simulink model "EMB_M17"  (R2017b)
settings: Solver=VariableStepAuto  StartTime=0.0  StopTime=10.0  RelTol=1e-3
undefined symbols (not defined in the file): a, b, c_break, c_gear, D_Kraft, D_Pos, d_rot, d_trans, i, I_Kraft, I_Pos, J, K, L, m, P_Kraft, P_Pos, R, t0, t1, T_abtast, x0, x_break
libraries: simulink x4

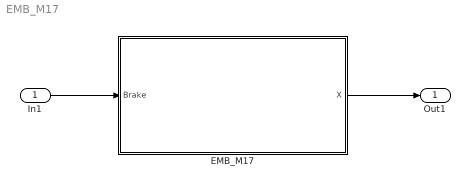
== system EMB_M17 ==
  In1 : Inport
  EMB_M17 : Subsystem
  Out1 : Outport
  wires:
  EMB_M17/1(X) -> Out1/1
  In1/1 -> EMB_M17/1(Brake)

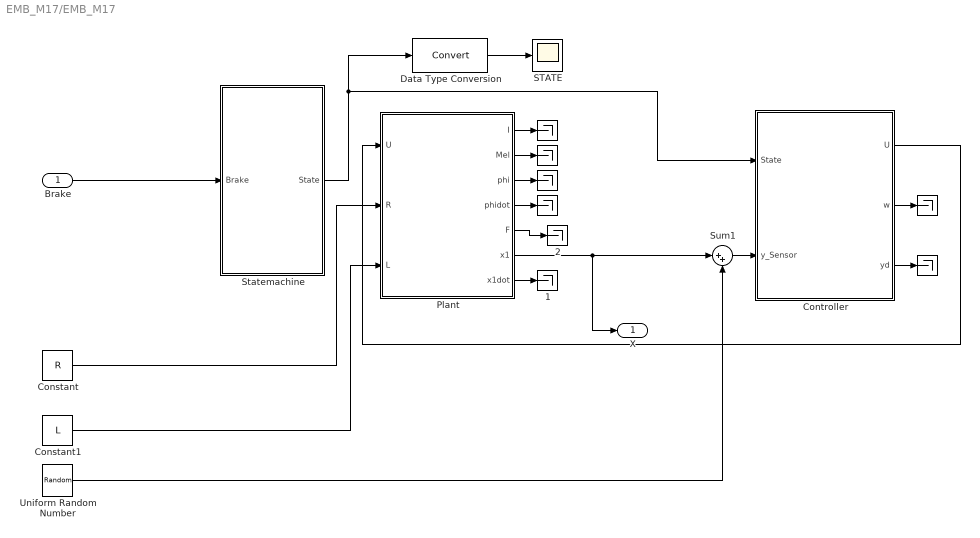
== system EMB_M17/EMB_M17 ==
  Brake : Inport
  "  " : Terminator
  "   " : Terminator
  "    " : Terminator
  "      " : Terminator
  "        " : Terminator
  "          " : Terminator
  "   1" : Terminator
  "   2" : Terminator
  Constant : Constant  Value=R
  Constant1 : Constant  Value=L
  Controller : Subsystem
  Data Type Conversion : DataTypeConversion
  Plant : Subsystem
  STATE : Scope
  Statemachine : Subsystem
  Sum1 : Sum  Inputs=|++
  Uniform Random Number : UniformRandomNumber  Minimum=-0.05  Maximum=0.05  SampleTime=0.000005
  X : Outport
  wires:
  Constant1/1 -> Plant/3(L)
  Constant/1 -> Plant/2(R)
  Data Type Conversion/1 -> STATE/1
  Statemachine/1(State) -> Data Type Conversion/1, Controller/1(State)
  Controller/3(yd) -> "        "/1
  Controller/2(w) -> "          "/1
  Controller/1(U) -> Plant/1(U)
  Sum1/1 -> Controller/2(y_Sensor)
  Plant/1(I) -> "      "/1
  Plant/2(Mel) -> "    "/1
  Uniform Random Number/1 -> Sum1/2
  Plant/7(x1dot) -> "   1"/1
  Plant/5(F) -> "   2"/1
  Plant/4(phidot) -> "   "/1
  Plant/3(phi) -> "  "/1
  Plant/6(x1) -> Sum1/1, X/1
  Brake/1 -> Statemachine/1(Brake)

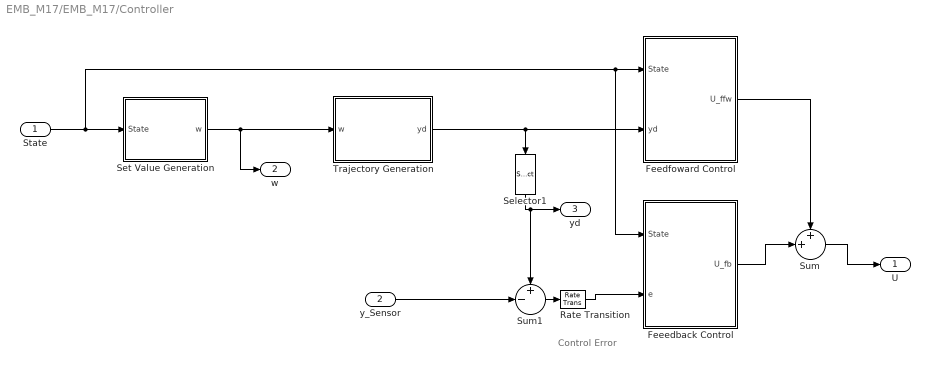
== system EMB_M17/EMB_M17/Controller ==
  note: Control Error
  State : Inport
  y_Sensor : Inport  Port=2
  Feedfoward Control : Subsystem
  Feeedback Control : Subsystem
  Rate Transition : RateTransition
  Selector1 : Selector  InputPortWidth=6  IndexOptions=Index vector (dialog)  Indices=[1]  OutputSizes=1
  Set Value Generation : Subsystem
  Sum : Sum  Inputs=++|
  Sum1 : Sum  Inputs=+-|
  Trajectory Generation : Subsystem
  U : Outport
  w : Outport  Port=2
  yd : Outport  Port=3
  wires:
  Rate Transition/1 -> Feeedback Control/2(e)
  y_Sensor/1 -> Sum1/2
  Selector1/1 -> yd/1, Sum1/1
  Sum1/1 -> Rate Transition/1
  Feeedback Control/1(U_fb) -> Sum/2
  Sum/1 -> U/1
  Feedfoward Control/1(U_ffw) -> Sum/1
  Trajectory Generation/1(yd) -> Selector1/1, Feedfoward Control/2(yd)
  Set Value Generation/1(w) -> w/1, Trajectory Generation/1(w)
  State/1 -> Feeedback Control/1(State), Feedfoward Control/1(State), Set Value Generation/1(State)

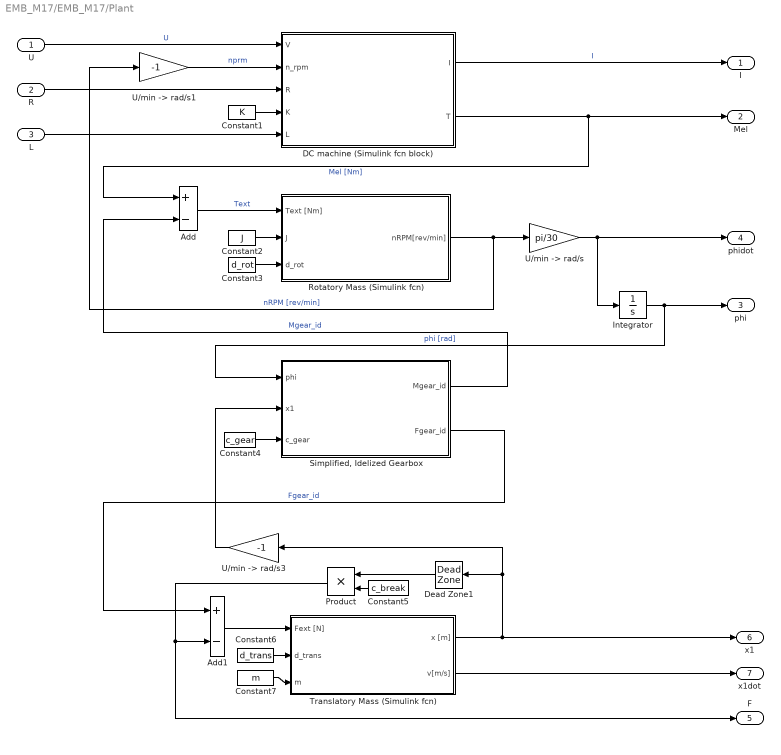
== system EMB_M17/EMB_M17/Plant ==
  U : Inport
  R : Inport  Port=2
  L : Inport  Port=3
  Add : Sum  Inputs=+-
  Add1 : Sum  Inputs=+-
  Constant1 : Constant  Value=K
  Constant2 : Constant  Value=J
  Constant3 : Constant  Value=d_rot
  Constant4 : Constant  Value=c_gear
  Constant5 : Constant  Value=c_break
  Constant6 : Constant  Value=d_trans
  Constant7 : Constant  Value=m
  DC machine (Simulink fcn block) : Subsystem
  Dead Zone1 : DeadZone  LowerValue=-inf  UpperValue=x0  SaturateOnIntegerOverflow=on
  Integrator : Integrator
  Product : Product
  Rotatory Mass (Simulink fcn) : Subsystem
  "Simplified, Idelized Gearbox" : Subsystem
  Translatory Mass (Simulink fcn) : Subsystem
  "U/min -> rad/s" : Gain  Gain=pi/30
  "U/min -> rad/s1" : Gain  Gain=-1
  "U/min -> rad/s3" : Gain  Gain=-1
  I : Outport
  Mel : Outport  Port=2
  phi : Outport  Port=3
  phidot : Outport  Port=4
  F : Outport  Port=5
  x1 : Outport  Port=6
  x1dot : Outport  Port=7
  wires:
  Constant7/1 -> Translatory Mass (Simulink fcn)/3(m)
  Constant6/1 -> Translatory Mass (Simulink fcn)/2(d_trans)
  Constant5/1 -> Product/2
  Constant4/1 -> "Simplified, Idelized Gearbox"/3(c_gear)
  Constant3/1 -> Rotatory Mass (Simulink fcn)/3(d_rot)
  Constant2/1 -> Rotatory Mass (Simulink fcn)/2(J)
  L/1 -> DC machine (Simulink fcn block)/5(L)
  Constant1/1 -> DC machine (Simulink fcn block)/4(K)
  R/1 -> DC machine (Simulink fcn block)/3(R)
  Translatory Mass (Simulink fcn)/2(v[m/s]) -> x1dot/1
  DC machine (Simulink fcn block)/1(I) -> I/1  "I"
  Add/1 -> Rotatory Mass (Simulink fcn)/1(Text [Nm])  "Text"
  Rotatory Mass (Simulink fcn)/1(nRPM[rev/min]) -> "U/min -> rad/s1"/1, "U/min -> rad/s"/1  "nRPM [rev/min]"
  "U/min -> rad/s"/1 -> phidot/1, Integrator/1
  Integrator/1 -> "Simplified, Idelized Gearbox"/1(phi), phi/1  "phi [rad]"
  Add1/1 -> Translatory Mass (Simulink fcn)/1(Fext [N])
  Translatory Mass (Simulink fcn)/1(x [m]) -> x1/1, "U/min -> rad/s3"/1, Dead Zone1/1
  DC machine (Simulink fcn block)/2(T) -> Add/1, Mel/1  "Mel [Nm]"
  "Simplified, Idelized Gearbox"/1(Mgear_id) -> Add/2  "Mgear_id"
  "Simplified, Idelized Gearbox"/2(Fgear_id) -> Add1/1  "Fgear_id"
  "U/min -> rad/s3"/1 -> "Simplified, Idelized Gearbox"/2(x1)
  Dead Zone1/1 -> Product/1
  Product/1 -> Add1/2, F/1
  "U/min -> rad/s1"/1 -> DC machine (Simulink fcn block)/2(n_rpm)  "nprm"
  U/1 -> DC machine (Simulink fcn block)/1(V)  "U"

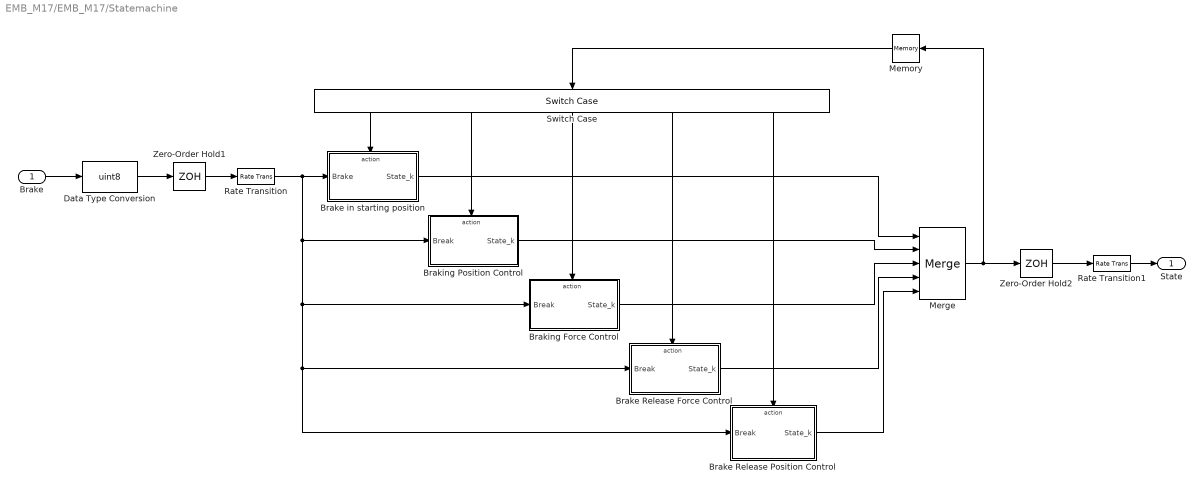
== system EMB_M17/EMB_M17/Statemachine ==
  Brake : Inport
  Brake Release Force Control : Subsystem  TreatAsAtomicUnit=on
  Brake Release Position Control : Subsystem  TreatAsAtomicUnit=on
  Brake in starting position : Subsystem  TreatAsAtomicUnit=on
  Braking Force Control : Subsystem  TreatAsAtomicUnit=on
  Braking Position Control : Subsystem  TreatAsAtomicUnit=on
  Data Type Conversion : DataTypeConversion  OutDataTypeStr=uint8
  Memory : Memory  InheritSampleTime=on
  Merge : Merge  Inputs=5  InitialOutput=0
  Rate Transition : RateTransition
  Rate Transition1 : RateTransition
  Switch Case : SwitchCase  CaseConditions={0,1,2,3,4}  ShowDefaultCase=off
  Zero-Order Hold1 : ZeroOrderHold  SampleTime=T_abtast
  Zero-Order Hold2 : ZeroOrderHold  SampleTime=T_abtast
  State : Outport
  wires:
  Rate Transition1/1 -> State/1
  Rate Transition/1 -> Brake Release Position Control/1(Break), Brake Release Force Control/1(Break), Braking Force Control/1(Break), Braking Position Control/1(Break), Brake in starting position/1(Brake)
  Brake/1 -> Data Type Conversion/1
  Data Type Conversion/1 -> Zero-Order Hold1/1
  Zero-Order Hold2/1 -> Rate Transition1/1
  Brake Release Position Control/1(State_k) -> Merge/5
  Brake Release Force Control/1(State_k) -> Merge/4
  Braking Force Control/1(State_k) -> Merge/3
  Braking Position Control/1(State_k) -> Merge/2
  Brake in starting position/1(State_k) -> Merge/1
  Switch Case/5 -> Brake Release Position Control/Action
  Switch Case/4 -> Brake Release Force Control/Action
  Switch Case/3 -> Braking Force Control/Action
  Switch Case/2 -> Braking Position Control/Action
  Switch Case/1 -> Brake in starting position/Action
  Zero-Order Hold1/1 -> Rate Transition/1
  Memory/1 -> Switch Case/1
  Merge/1 -> Zero-Order Hold2/1, Memory/1

== system EMB_M17/EMB_M17/Controller/Feedfoward Control ==
  State : Inport
  yd : Inport  Port=2
  Constant : Constant  Value=0
  Demux : Demux  Outputs=6
  Feedforward Control Force : S-Function  FunctionName=InverseEMBforce  Parameters=R,L,K,J,dvrot,m,dvtrans,cgear,i,cbreak,x0,xic  SFunctionDeploymentMode=off  EnableBusSupport=off  mask{R=R, L=L, K=K, J=J, dvrot=d_rot, m=m, dvtrans=d_trans, cgear=c_gear, i=i, cbreak=c_break, x0=x0, xic=[0]}
      mask prompts: R "Widerstand R [Ohm]:"; L "Induktivitaet L [H]:"; K "Motorkonstante K [Vs]:"; J "Traegheitsmoment J [kgm^2]:"; dvrot "Viskose Reibung dvrot [Nms/rad]:"; m "Masse m [kg]:"; dvtrans "Viskose Reibung dvtrans [Ns/m]:"; cgear "Steifigkeit Getriebe cgear [N/m]:"; i "Uebersetzung i [-]:"; cbreak "Steifigkeit Bremse cbreak [N/m]:"; x0 "Position x0 [m]:"; xic "Vector of continuous initial conditions [Initial Dummy]"
  Feedforward Control Position : Fcn  Expr="(a(1)*u[6] + a(2)*u[5] + a(3)*u[4] + a(4)*u[3]  + a(5)*u[2] + a(6)*u[1] )/b"
  Multiport Switch : MultiPortSwitch  DataPortOrder=Zero-based contiguous  Inputs=5  zeroidx=on
  U_ffw : Outport
  wires:
  Multiport Switch/1 -> U_ffw/1
  Feedforward Control Force/1 -> Multiport Switch/5, Multiport Switch/4
  Feedforward Control Position/1 -> Multiport Switch/6, Multiport Switch/3
  Constant/1 -> Multiport Switch/2
  Demux/6 -> Feedforward Control Force/6
  Demux/5 -> Feedforward Control Force/5
  Demux/4 -> Feedforward Control Force/4
  Demux/3 -> Feedforward Control Force/3
  Demux/2 -> Feedforward Control Force/2
  Demux/1 -> Feedforward Control Force/1
  yd/1 -> Demux/1, Feedforward Control Position/1
  State/1 -> Multiport Switch/1

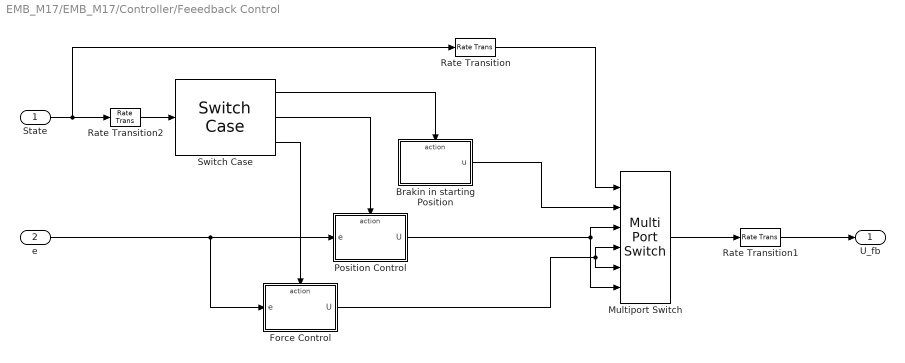
== system EMB_M17/EMB_M17/Controller/Feeedback Control ==
  State : Inport
  e : Inport  Port=2
  Brakin in starting Position : Subsystem  TreatAsAtomicUnit=on
  Force Control : Subsystem  TreatAsAtomicUnit=on
  Multiport Switch : MultiPortSwitch  DataPortOrder=Zero-based contiguous  Inputs=5  zeroidx=on
  Position Control : Subsystem  TreatAsAtomicUnit=on
  Rate Transition : RateTransition
  Rate Transition1 : RateTransition
  Rate Transition2 : RateTransition
  Switch Case : SwitchCase  CaseConditions={0,[1,4],[2,3]}  ShowDefaultCase=off  SampleTime=T_abtast
  U_fb : Outport
  wires:
  Rate Transition2/1 -> Switch Case/1
  Rate Transition1/1 -> U_fb/1
  Rate Transition/1 -> Multiport Switch/1
  Multiport Switch/1 -> Rate Transition1/1
  Force Control/1(U) -> Multiport Switch/5, Multiport Switch/4
  Brakin in starting Position/1(u) -> Multiport Switch/2
  Position Control/1(U) -> Multiport Switch/6, Multiport Switch/3
  Switch Case/3 -> Force Control/Action
  Switch Case/2 -> Position Control/Action
  e/1 -> Force Control/1(e), Position Control/1(e)
  Switch Case/1 -> Brakin in starting Position/Action
  State/1 -> Rate Transition/1, Rate Transition2/1

== system EMB_M17/EMB_M17/Controller/Set Value Generation ==
  State : Inport
  Brake Release Force control : Subsystem  TreatAsAtomicUnit=on
  Brake Release Position Control : Subsystem  TreatAsAtomicUnit=on
  Brake in starting position : Subsystem  TreatAsAtomicUnit=on
  Braking Force control : Subsystem  TreatAsAtomicUnit=on
  Braking Position Control : Subsystem  TreatAsAtomicUnit=on
  Merge : Merge  Inputs=5  InitialOutput=0
  Switch Set Value : SwitchCase  CaseConditions={0,1,2,3,4}  ShowDefaultCase=off
  w : Outport
  wires:
  Merge/1 -> w/1
  State/1 -> Switch Set Value/1
  Brake Release Position Control/1(u) -> Merge/5
  Switch Set Value/5 -> Brake Release Position Control/Action
  Brake Release Force control/1(u) -> Merge/4
  Braking Force control/1(u) -> Merge/3
  Switch Set Value/4 -> Brake Release Force control/Action
  Switch Set Value/3 -> Braking Force control/Action
  Braking Position Control/1(u) -> Merge/2
  Switch Set Value/2 -> Braking Position Control/Action
  Brake in starting position/1(u) -> Merge/1
  Switch Set Value/1 -> Brake in starting position/Action

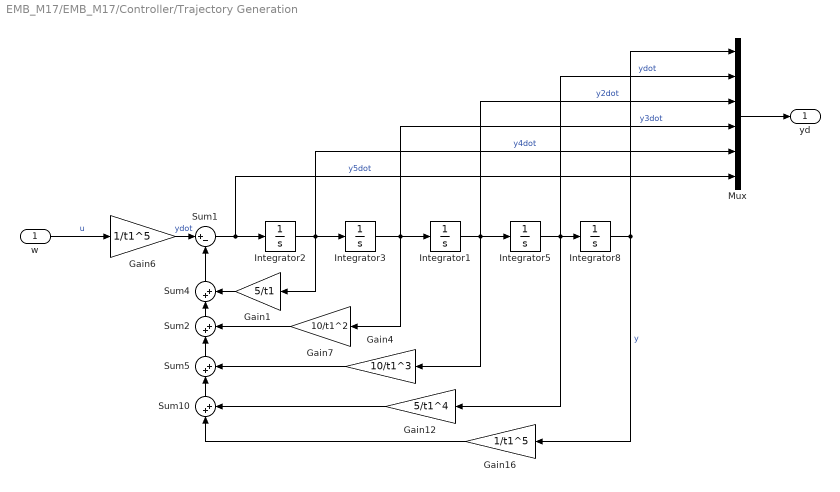
== system EMB_M17/EMB_M17/Controller/Trajectory Generation ==
  w : Inport
  Gain1 : Gain  Gain=5/t1
  Gain12 : Gain  Gain=5/t1^4
  Gain16 : Gain  Gain=1/t1^5
  Gain4 : Gain  Gain=10/t1^3
  Gain6 : Gain  Gain=1/t1^5
  Gain7 : Gain  Gain=10/t1^2
  Integrator{1..3,5,8} (5 alike) : Integrator
  Mux : Mux  Inputs=6
  Sum1 : Sum  Inputs=|+-
  Sum{2,4..5,10} (4 alike) : Sum  Inputs=|++
  yd : Outport
  wires:
  Gain16/1 -> Sum10/1
  Sum10/1 -> Sum5/1
  Gain12/1 -> Sum10/2
  Integrator8/1 -> Mux/1, Gain16/1  "y"
  Sum5/1 -> Sum2/1
  Integrator5/1 -> Integrator8/1, Mux/2, Gain12/1  "ydot"
  Sum2/1 -> Sum4/1
  Gain1/1 -> Sum4/2
  Sum4/1 -> Sum1/2
  Gain4/1 -> Sum5/2
  Integrator1/1 -> Integrator5/1, Mux/3, Gain4/1  "y2dot"
  Gain7/1 -> Sum2/2
  Integrator3/1 -> Integrator1/1, Mux/4, Gain7/1  "y3dot"
  Gain6/1 -> Sum1/1  "ydot"
  Sum1/1 -> Mux/6, Integrator2/1  "y5dot"
  Integrator2/1 -> Integrator3/1, Mux/5, Gain1/1  "y4dot"
  Mux/1 -> yd/1
  w/1 -> Gain6/1  "u"

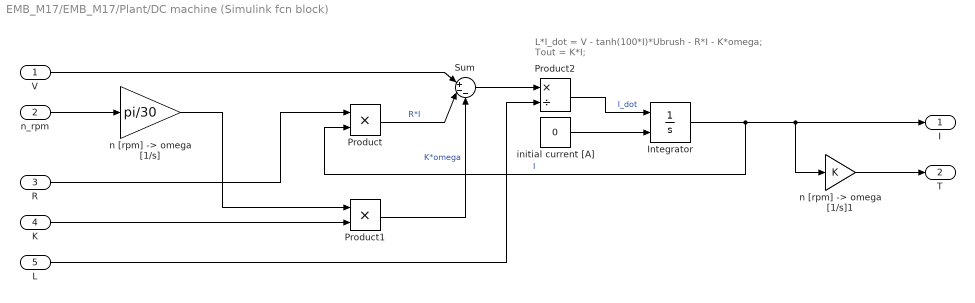
== system EMB_M17/EMB_M17/Plant/DC machine (Simulink fcn block) ==
  note: L*I_dot = V - tanh(100*I)*Ubrush - R*I - K*omega;
      | Tout = K*I;
  V : Inport
  n_rpm : Inport  Port=2
  R : Inport  Port=3
  K : Inport  Port=4
  L : Inport  Port=5
  Integrator : Integrator  InitialConditionSource=external
  Product : Product
  Product1 : Product
  Product2 : Product  Inputs=*/
  Sum : Sum  Inputs=|+--
  initial current [A] : Constant  Value=0
  "n [rpm] -> omega [1/s]" : Gain  Gain=pi/30
  "n [rpm] -> omega [1/s]1" : Gain  Gain=K
  I : Outport
  T : Outport  Port=2
  wires:
  Sum/1 -> Product2/1
  L/1 -> Product2/2
  K/1 -> Product1/2
  Product1/1 -> Sum/3  "K*omega"
  Product/1 -> Sum/2  "R*I"
  R/1 -> Product/1
  initial current [A]/1 -> Integrator/2
  Integrator/1 -> "n [rpm] -> omega [1/s]1"/1, I/1, Product/2  "I"
  Product2/1 -> Integrator/1  "I_dot"
  "n [rpm] -> omega [1/s]1"/1 -> T/1
  "n [rpm] -> omega [1/s]"/1 -> Product1/1
  V/1 -> Sum/1
  n_rpm/1 -> "n [rpm] -> omega [1/s]"/1

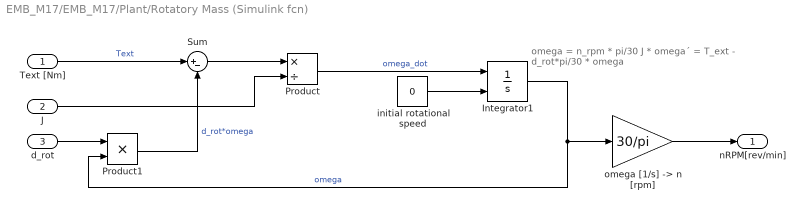
== system EMB_M17/EMB_M17/Plant/Rotatory Mass (Simulink fcn) ==
  note: omega = n_rpm * pi/30
      |
      | J * omega´ = T_ext -  d_rot*pi/30 * omega
  Text [Nm] : Inport
  J : Inport  Port=2
  d_rot : Inport  Port=3
  Integrator1 : Integrator  InitialConditionSource=external
  Product : Product  Inputs=*/
  Product1 : Product
  Sum : Sum  Inputs=|+-
  initial rotational speed : Constant  Value=0
  "omega [1/s] -> n [rpm]" : Gain  Gain=30/pi
  nRPM[rev/min] : Outport
  wires:
  Sum/1 -> Product/1
  d_rot/1 -> Product1/1
  Text [Nm]/1 -> Sum/1  "Text"
  Product1/1 -> Sum/2  "d_rot*omega"
  J/1 -> Product/2
  Integrator1/1 -> "omega [1/s] -> n [rpm]"/1, Product1/2  "omega"
  initial rotational speed/1 -> Integrator1/2
  Product/1 -> Integrator1/1  "omega_dot"
  "omega [1/s] -> n [rpm]"/1 -> nRPM[rev/min]/1

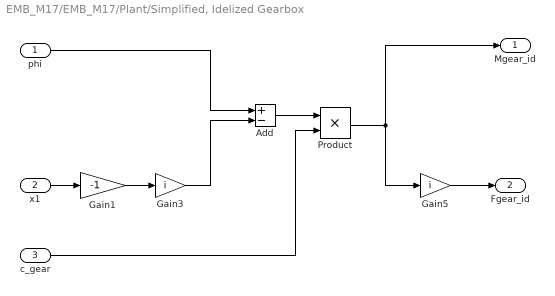
== system EMB_M17/EMB_M17/Plant/Simplified, Idelized Gearbox ==
  phi : Inport
  x1 : Inport  Port=2
  c_gear : Inport  Port=3
  Add : Sum  Inputs=+-
  Gain1 : Gain  Gain=-1
  Gain3 : Gain  Gain=i
  Gain5 : Gain  Gain=i
  Product : Product
  Mgear_id : Outport
  Fgear_id : Outport  Port=2
  wires:
  c_gear/1 -> Product/2
  phi/1 -> Add/1
  Gain3/1 -> Add/2
  Add/1 -> Product/1
  Product/1 -> Gain5/1, Mgear_id/1
  Gain5/1 -> Fgear_id/1
  x1/1 -> Gain1/1
  Gain1/1 -> Gain3/1

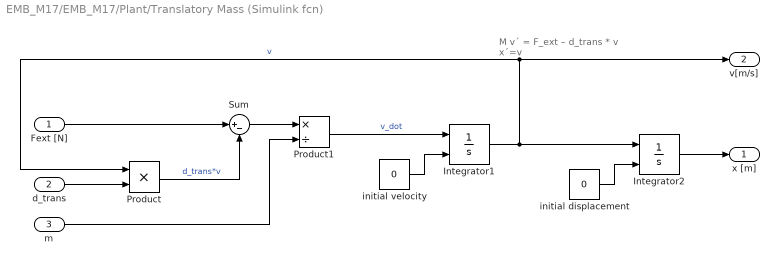
== system EMB_M17/EMB_M17/Plant/Translatory Mass (Simulink fcn) ==
  note: M v´ = F_ext – d_trans * v
      |
      | x´=v
  Fext [N] : Inport
  d_trans : Inport  Port=2
  m : Inport  Port=3
  Integrator1 : Integrator  InitialConditionSource=external
  Integrator2 : Integrator  InitialConditionSource=external
  Product : Product
  Product1 : Product  Inputs=*/
  Sum : Sum  Inputs=|+-
  initial displacement : Constant  Value=0
  "initial velocity " : Constant  Value=0
  x [m] : Outport
  v[m/s] : Outport  Port=2
  wires:
  m/1 -> Product1/2
  Sum/1 -> Product1/1
  Product/1 -> Sum/2  "d_trans*v"
  d_trans/1 -> Product/2
  Integrator2/1 -> x [m]/1
  Product1/1 -> Integrator1/1  "v_dot"
  "initial velocity "/1 -> Integrator1/2
  Integrator1/1 -> Integrator2/1, Product/1, v[m/s]/1  "v"
  Fext [N]/1 -> Sum/1
  initial displacement/1 -> Integrator2/2

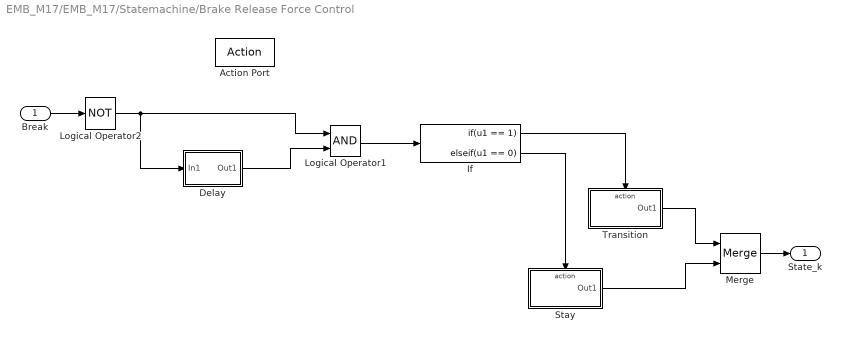
== system EMB_M17/EMB_M17/Statemachine/Brake Release Force Control ==
  Break : Inport
  Action Port : ActionPort  InitializeStates=reset
  Delay : Subsystem
  If : If  IfExpression=u1 == 1  ElseIfExpressions=u1 == 0  ShowElse=off
  Logical Operator1 : Logic  AllPortsSameDT=off  OutDataTypeStr=boolean
  Logical Operator2 : Logic  Operator=NOT  AllPortsSameDT=off  OutDataTypeStr=boolean
  Merge : Merge
  Stay : Subsystem  TreatAsAtomicUnit=on
  Transition : Subsystem  TreatAsAtomicUnit=on
  State_k : Outport
  wires:
  Delay/1(Out1) -> Logical Operator1/2
  Logical Operator2/1 -> Delay/1(In1), Logical Operator1/1
  Logical Operator1/1 -> If/1
  Break/1 -> Logical Operator2/1
  If/1 -> Transition/Action
  If/2 -> Stay/Action
  Transition/1(Out1) -> Merge/1
  Stay/1(Out1) -> Merge/2
  Merge/1 -> State_k/1

== system EMB_M17/EMB_M17/Statemachine/Brake Release Position Control ==
  Break : Inport
  Action Port : ActionPort  InitializeStates=reset
  Delay : Subsystem
  If : If  IfExpression=u1 == 1  ElseIfExpressions=u1 == 0  ShowElse=off
  Logical Operator1 : Logic  Operator=NOR  AllPortsSameDT=off  OutDataTypeStr=boolean
  Logical Operator2 : Logic  Operator=NOT  AllPortsSameDT=off  OutDataTypeStr=boolean
  Merge : Merge
  Stay : Subsystem  TreatAsAtomicUnit=on
  Transition : Subsystem  TreatAsAtomicUnit=on
  State_k : Outport
  wires:
  Delay/1(Out1) -> Logical Operator1/2
  Logical Operator2/1 -> Delay/1(In1), Logical Operator1/1
  Logical Operator1/1 -> If/1
  Break/1 -> Logical Operator2/1
  If/1 -> Transition/Action
  If/2 -> Stay/Action
  Transition/1(Out1) -> Merge/1
  Stay/1(Out1) -> Merge/2
  Merge/1 -> State_k/1

== system EMB_M17/EMB_M17/Statemachine/Brake in starting position ==
  Brake : Inport
  Action Port : ActionPort
  If : If  IfExpression=u1 == 1  ElseIfExpressions=u1 == 0  ShowElse=off
  Merge : Merge
  Stay : Subsystem  TreatAsAtomicUnit=on
  Transition : Subsystem  TreatAsAtomicUnit=on
  State_k : Outport
  wires:
  Merge/1 -> State_k/1
  Stay/1(Out1) -> Merge/2
  Transition/1(Out1) -> Merge/1
  If/2 -> Stay/Action
  If/1 -> Transition/Action
  Brake/1 -> If/1

== system EMB_M17/EMB_M17/Statemachine/Braking Force Control ==
  Break : Inport
  Action Port : ActionPort
  If : If  IfExpression=u1 == 0  ElseIfExpressions=u1 == 1  ShowElse=off
  Merge : Merge
  Stay : Subsystem  TreatAsAtomicUnit=on
  Transition : Subsystem  TreatAsAtomicUnit=on
  State_k : Outport
  wires:
  Break/1 -> If/1
  If/1 -> Transition/Action
  If/2 -> Stay/Action
  Transition/1(Out1) -> Merge/1
  Stay/1(Out1) -> Merge/2
  Merge/1 -> State_k/1

== system EMB_M17/EMB_M17/Statemachine/Braking Position Control ==
  Break : Inport
  Action Port : ActionPort  InitializeStates=reset
  Delay : Subsystem
  Delay1 : Subsystem
  If : If  IfExpression=u1 == 1  ElseIfExpressions=u1 == 0  ShowElse=off
  Logical Operator : Logic  AllPortsSameDT=off  OutDataTypeStr=boolean
  Merge : Merge
  Stay : Subsystem  TreatAsAtomicUnit=on
  Transition : Subsystem  TreatAsAtomicUnit=on
  State_k : Outport
  wires:
  Delay/1(Out1) -> Logical Operator/2
  Logical Operator/1 -> If/1
  Break/1 -> Delay1/1(In1), Logical Operator/1
  Merge/1 -> State_k/1
  Stay/1(Out1) -> Merge/2
  Transition/1(Out1) -> Merge/1
  If/2 -> Stay/Action
  If/1 -> Transition/Action
  Delay1/1(Out1) -> Delay/1(In1)

== system EMB_M17/EMB_M17/Controller/Feeedback Control/Brakin in starting Position ==
  Action Port : ActionPort
  Constant : Constant  Value=0
  u : Outport  SourceOfInitialOutputValue=Input signal
  wires:
  Constant/1 -> u/1

== system EMB_M17/EMB_M17/Controller/Feeedback Control/Force Control ==
  e : Inport
  Action Port : ActionPort  InitializeStates=reset
  Gain : Gain
  PIDT1 zeitdiskret : Subsystem
  U : Outport  InitialOutput=0
  wires:
  e/1 -> PIDT1 zeitdiskret/1(u)
  PIDT1 zeitdiskret/1(y) -> Gain/1
  Gain/1 -> U/1

== system EMB_M17/EMB_M17/Controller/Feeedback Control/Position Control ==
  e : Inport
  Action Port : ActionPort  InitializeStates=reset
  Gain : Gain
  PIDT1 zeitdiskret : Subsystem
  U : Outport  InitialOutput=0
  wires:
  Gain/1 -> U/1
  PIDT1 zeitdiskret/1(y) -> Gain/1
  e/1 -> PIDT1 zeitdiskret/1(u)

== system EMB_M17/EMB_M17/Controller/Set Value Generation/Brake Release Force control ==
  Action Port : ActionPort
  Constant : Constant  Value=x0
  u : Outport
  wires:
  Constant/1 -> u/1

== system EMB_M17/EMB_M17/Controller/Set Value Generation/Brake Release Position Control ==
  Action Port : ActionPort
  Constant : Constant  Value=0
  u : Outport
  wires:
  Constant/1 -> u/1

== system EMB_M17/EMB_M17/Controller/Set Value Generation/Brake in starting position ==
  Action Port : ActionPort
  Constant : Constant  Value=0
  u : Outport
  wires:
  Constant/1 -> u/1

== system EMB_M17/EMB_M17/Controller/Set Value Generation/Braking Force control ==
  Action Port : ActionPort
  Constant : Constant  Value=x0 + x_break
  u : Outport
  wires:
  Constant/1 -> u/1

== system EMB_M17/EMB_M17/Controller/Set Value Generation/Braking Position Control ==
  Action Port : ActionPort
  Constant : Constant  Value=x0
  u : Outport
  wires:
  Constant/1 -> u/1

== system EMB_M17/EMB_M17/Statemachine/Brake Release Force Control/Delay ==
  In1 : Inport
  Compare To Constant : simulink/Logic and Bit Operations/Compare To Constant  relop=>=  const=t0  OutDataTypeStr=uint8  ZeroCross=off
  Data Type Conversion : DataTypeConversion
  Integrator : Integrator
  Out1 : Outport
  wires:
  Data Type Conversion/1 -> Integrator/1
  Compare To Constant/1 -> Out1/1
  Integrator/1 -> Compare To Constant/1
  In1/1 -> Data Type Conversion/1

== system EMB_M17/EMB_M17/Statemachine/Brake Release Force Control/Stay ==
  Action Port : ActionPort
  Constant : Constant  Value=3  OutDataTypeStr=uint8
  Out1 : Outport
  wires:
  Constant/1 -> Out1/1

== system EMB_M17/EMB_M17/Statemachine/Brake Release Force Control/Transition ==
  Action Port : ActionPort
  Constant : Constant  Value=4  OutDataTypeStr=uint8
  Out1 : Outport
  wires:
  Constant/1 -> Out1/1

== system EMB_M17/EMB_M17/Statemachine/Brake Release Position Control/Delay ==
  In1 : Inport
  Compare To Constant : simulink/Logic and Bit Operations/Compare To Constant  relop=>=  const=t0  OutDataTypeStr=uint8  ZeroCross=off
  Data Type Conversion : DataTypeConversion
  Integrator : Integrator
  Out1 : Outport
  wires:
  Data Type Conversion/1 -> Integrator/1
  Compare To Constant/1 -> Out1/1
  Integrator/1 -> Compare To Constant/1
  In1/1 -> Data Type Conversion/1

== system EMB_M17/EMB_M17/Statemachine/Brake Release Position Control/Stay ==
  Action Port : ActionPort
  Constant : Constant  Value=4  OutDataTypeStr=uint8
  Out1 : Outport
  wires:
  Constant/1 -> Out1/1

== system EMB_M17/EMB_M17/Statemachine/Brake Release Position Control/Transition ==
  Action Port : ActionPort
  Constant : Constant  Value=0  OutDataTypeStr=uint8
  Out1 : Outport
  wires:
  Constant/1 -> Out1/1

== system EMB_M17/EMB_M17/Statemachine/Brake in starting position/Stay ==
  Action Port : ActionPort
  Constant : Constant  Value=0  OutDataTypeStr=uint8
  Out1 : Outport
  wires:
  Constant/1 -> Out1/1

== system EMB_M17/EMB_M17/Statemachine/Brake in starting position/Transition ==
  Action Port : ActionPort
  Constant : Constant  OutDataTypeStr=uint8
  Out1 : Outport
  wires:
  Constant/1 -> Out1/1

== system EMB_M17/EMB_M17/Statemachine/Braking Force Control/Stay ==
  Action Port : ActionPort
  Constant : Constant  Value=2  OutDataTypeStr=uint8
  Out1 : Outport
  wires:
  Constant/1 -> Out1/1

== system EMB_M17/EMB_M17/Statemachine/Braking Force Control/Transition ==
  Action Port : ActionPort
  Constant : Constant  Value=3  OutDataTypeStr=uint8
  Out1 : Outport
  wires:
  Constant/1 -> Out1/1

== system EMB_M17/EMB_M17/Statemachine/Braking Position Control/Delay ==
  In1 : Inport
  Compare To Constant : simulink/Logic and Bit Operations/Compare To Constant  relop=>=  const=t0  OutDataTypeStr=uint8  ZeroCross=off
  Data Type Conversion : DataTypeConversion
  Integrator : Integrator
  Out1 : Outport
  wires:
  Data Type Conversion/1 -> Integrator/1
  Compare To Constant/1 -> Out1/1
  Integrator/1 -> Compare To Constant/1
  In1/1 -> Data Type Conversion/1

== system EMB_M17/EMB_M17/Statemachine/Braking Position Control/Delay1 ==
  In1 : Inport
  Compare To Constant : simulink/Logic and Bit Operations/Compare To Constant  relop=>=  const=t0  OutDataTypeStr=uint8  ZeroCross=off
  Data Type Conversion : DataTypeConversion
  Integrator : Integrator
  Out1 : Outport
  wires:
  In1/1 -> Data Type Conversion/1
  Integrator/1 -> Compare To Constant/1
  Compare To Constant/1 -> Out1/1
  Data Type Conversion/1 -> Integrator/1

== system EMB_M17/EMB_M17/Statemachine/Braking Position Control/Stay ==
  Action Port : ActionPort
  Constant : Constant  OutDataTypeStr=uint8
  Out1 : Outport
  wires:
  Constant/1 -> Out1/1

== system EMB_M17/EMB_M17/Statemachine/Braking Position Control/Transition ==
  Action Port : ActionPort
  Constant : Constant  Value=2  OutDataTypeStr=uint8
  Out1 : Outport
  wires:
  Constant/1 -> Out1/1

== system EMB_M17/EMB_M17/Controller/Feeedback Control/Force Control/PIDT1 zeitdiskret ==
  u : Inport
  Discrete Transfer Fcn : DiscreteTransferFcn  Numerator=[1 1]  Denominator=[1 -1]  SampleTime=T_abtast
  Discrete Transfer Fcn1 : DiscreteTransferFcn  Numerator=[1 -1]  Denominator=[1+1/tan(T_abtast/2/1e-3) 1-1/tan(T_abtast/2/1e-3)]  SampleTime=T_abtast
  Sum : Sum  Inputs=3
  proportinal part : Gain  Gain=P_Kraft
  proportinal part1 : Gain  Gain=I_Kraft*T_abtast/2
  proportinal part2 : Gain  Gain=2*D_Kraft/T_abtast
  y : Outport
  wires:
  proportinal part/1 -> Sum/1
  u/1 -> proportinal part/1, proportinal part2/1, proportinal part1/1
  proportinal part2/1 -> Discrete Transfer Fcn1/1
  proportinal part1/1 -> Discrete Transfer Fcn/1
  Discrete Transfer Fcn1/1 -> Sum/3
  Discrete Transfer Fcn/1 -> Sum/2
  Sum/1 -> y/1

== system EMB_M17/EMB_M17/Controller/Feeedback Control/Position Control/PIDT1 zeitdiskret ==
  u : Inport
  Discrete Transfer Fcn : DiscreteTransferFcn  Numerator=[1 1]  Denominator=[1 -1]  SampleTime=T_abtast
  Discrete Transfer Fcn1 : DiscreteTransferFcn  Numerator=[1 -1]  Denominator=[1+1/tan(T_abtast/2/1e-3) 1-1/tan(T_abtast/2/1e-3)]  SampleTime=T_abtast
  Sum : Sum  Inputs=3
  proportinal part : Gain  Gain=P_Pos
  proportinal part1 : Gain  Gain=I_Pos*T_abtast/2
  proportinal part2 : Gain  Gain=2*D_Pos/T_abtast
  y : Outport
  wires:
  proportinal part2/1 -> Discrete Transfer Fcn1/1
  proportinal part1/1 -> Discrete Transfer Fcn/1
  Discrete Transfer Fcn1/1 -> Sum/3
  Discrete Transfer Fcn/1 -> Sum/2
  u/1 -> proportinal part/1, proportinal part2/1, proportinal part1/1
  proportinal part/1 -> Sum/1
  Sum/1 -> y/1
